simulink model "La1b_w_controller"  (R2024b)
settings: Solver=VariableStepAuto  StartTime=0.0  StopTime=40  RelTol=1e-3
values from neighbouring files (symbols this model uses):
  b = 666.1*10^-6    (= 0.0006661)    [Lab1b.m]
  J = 0.0081    [Lab1b.m]
  K_e = 0.094    [Lab1b.m]
  K_t = 0.094    [Lab1b.m]
  La = 528e-6    (= 0.000528)    [Lab1b.m]
  Ra = 0.649    [Lab1b.m]
settings Model: Creator=camer  LastModifiedBy=camer

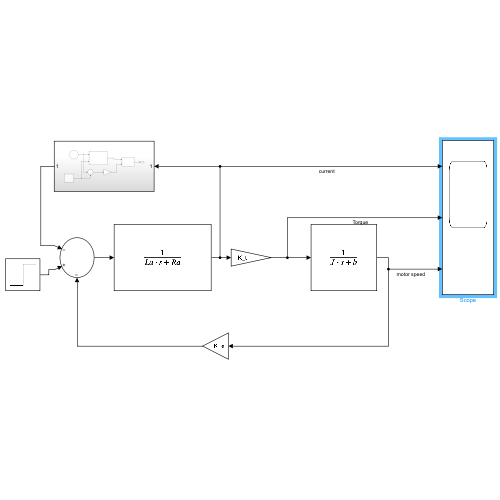
[thumbnail: Simulink's stored preview of the top-level diagram]
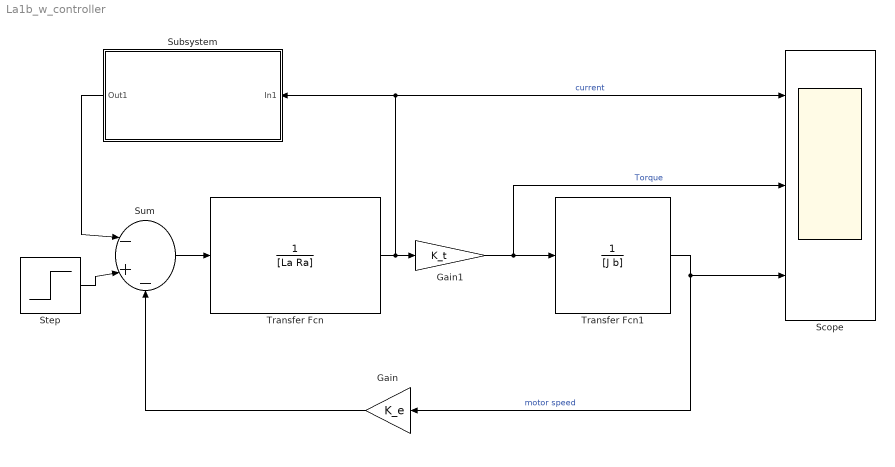
== system La1b_w_controller ==
  Gain : Gain  Gain=K_e
  Gain1 : Gain  Gain=K_t
  Scope : Scope  NumInputPorts=3
  Step : Step  After=60  SampleTime=0
  Subsystem : Subsystem
  Sum : Sum  Inputs=|-+-
  Transfer Fcn : TransferFcn  Denominator=[La Ra]
  Transfer Fcn1 : TransferFcn  Denominator=[J b]
  wires:
  Transfer Fcn1/1 -> Gain/1, Scope/3  "motor speed"
  Sum/1 -> Transfer Fcn/1
  Gain1/1 -> Scope/2, Transfer Fcn1/1  "Torque"
  Transfer Fcn/1 -> Subsystem/1(In1), Scope/1, Gain1/1  "current"
  Gain/1 -> Sum/3
  Step/1 -> Sum/2
  Subsystem/1(Out1) -> Sum/1

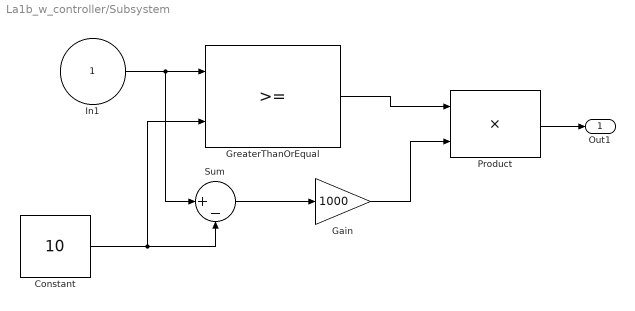
== system La1b_w_controller/Subsystem ==
  In1 : Inport
  Constant : Constant  Value=10
  Gain : Gain  Gain=1000
  GreaterThanOrEqual : RelationalOperator  OutDataTypeStr=boolean  RndMeth=Simplest  InputSameDT=off
  Product : Product
  Sum : Sum  Inputs=|+-
  Out1 : Outport
  wires:
  In1/1 -> Sum/1, GreaterThanOrEqual/1
  Constant/1 -> Sum/2, GreaterThanOrEqual/2
  Sum/1 -> Gain/1
  GreaterThanOrEqual/1 -> Product/1
  Gain/1 -> Product/2
  Product/1 -> Out1/1
